simulink model "Scenario_13_CoDeSys"  (R2012b)
settings: Solver=ode3  StartTime=0.0  StopTime=inf  FixedStep=Sample_Time_Model  RelTol=1e-3
PreLoadFcn:
  | Variablen_Scenario13
InitFcn:
  | BT = randperm(9);
values from neighbouring files (symbols this model uses):
  Band_Geschwindigkeit = 1.47    [Variablen_Scenario13.m]
  Band_Sensor_Hell_2_Z = -6.5    [Variablen_Scenario13.m]
  Band_Sensor_Hell_3_Z = -10.36    [Variablen_Scenario13.m]
  Band_Sensor_Hell_4_Z = -14.64    [Variablen_Scenario13.m]
  Band_Sensor_Tolerance_Z = 0.2    [Variablen_Scenario13.m]
  Bauteil_Fallgeschwindigkeit = 0.4    [Variablen_Scenario13.m]
  Bauteil_Farbe_Metall = [0.8 0.8 0.8]    [Variablen_Scenario13.m]
  Bauteil_Farbe_Schwarz = [0.2 0.2 0.2]    [Variablen_Scenario13.m]
  Bauteil_Farbe_Weiss = [1 1 0.2]    [Variablen_Scenario13.m]
  Kran_Dauer_90_Grad = 5    [Variablen_Scenario13.m]
  Kran_Drehwinkel_90_Grad = 8050    [Variablen_Scenario13.m]
  Kran_Sensor_Position_Delta = 0.07    [Variablen_Scenario13.m]
  Sample_Time_Model = 0.05    [Variablen_Scenario13.m]
  Sample_Time_Simulation = 0.1    [Variablen_Scenario13.m]
  Sensor_Band_Metall_1 = -6.5    [Variablen_Scenario13.m]
  Sensor_Band_Metall_2 = -10.36    [Variablen_Scenario13.m]
libraries: simulink x557, vrlib x13, opclib x7, rtwinlib x1
(part 4 of 10)

== stateflow chart Scenario_13_CoDeSys/Signal Expander/Bauteil_4 ==
  state Stop1
  state Bauteil_Pos_2
  state Bauteil_Unten
  state Bauteil_Pos_4
    entry:
    BT_X_Achse = 5.75;
    BT_Y_Achse = 3.75;
    x =0;
  state Bauteil_Faellt_3
    during:
    BT_Y_Achse = Next_Pos_Minus_Min(BT_Y_Achse, Bauteil_Fallgeschwindigkeit, 0.7);
  state Drehen_Rechts_Runter [function]
    (default) -> (junction 322) : {BT_Y_Achse = Next_Pos_Minus_Min(BT_Y_Achse, Kran_Zyl_Schritt_Runter, 0.65);
        | x = x - Kran_Drehen_Schritt;
        | BT_Z_Achse = -3.5*sin(x);
        | BT_X_Achse = 3.5*cos(x);}
  state Drehen_Rechts_Hoch [function]
    (default) -> (junction 325) : {BT_Y_Achse = Next_Pos_Plus_Max(BT_Y_Achse, Kran_Zyl_Schritt_Hoch, 1.65);
        | x = x - Kran_Drehen_Schritt;
        | BT_Z_Achse = -3.5*sin(x);
        | BT_X_Achse = 3.5*cos(x);}
  state Bauteil_Lager_Vereinz_Ausfahren
    during:
    BT_X_Achse = BT_X_Achse - Lager_Vereinzler_Schritt_Aus;
  state Bauteil_Lager_Bereit
    entry: BT_Bereit = 1;
    BT_X_Achse = 3.5;
  state Drehen_Links_Runter [function]
    (default) -> (junction 319) : {BT_Y_Achse = Next_Pos_Minus_Min(BT_Y_Achse, Kran_Zyl_Schritt_Runter, 0.65);
        | x = x + Kran_Drehen_Schritt;
        | BT_Z_Achse = -3.5*sin(x);
        | BT_X_Achse = 3.5*cos(x);}
  state Drehen_Links_Hoch [function]
    (default) -> (junction 309) : {BT_Y_Achse = Next_Pos_Plus_Max(BT_Y_Achse, Kran_Zyl_Schritt_Hoch, 1.65);
        | x = x + Kran_Drehen_Schritt;
        | BT_Z_Achse = -3.5*sin(x);
        | BT_X_Achse = 3.5*cos(x);}
  state Ausgabe = Next_Pos_Plus_Max(Achse, Schrittgroesse, MaxWert) [function]
    (default) -> (junction 249) : {Naechste_Position = Achse + Schrittgroesse;}
    (junction 249) -> (junction 250) [order 1] : [Naechste_Position >= MaxWert]
    (junction 249) -> (junction 251) [order 2] : {Ausgabe = Naechste_Position;}
    (junction 250) -> (junction 252) : {Ausgabe = MaxWert;}
    (junction 252) -> (junction 251)
  state Bauteil_Pos_3
  state Bauteil_Kran_Hochheben_Bereit
    entry: BT_Bereit = 1;
    Kran_Sauger_BT = 1;
  state Bauteil_Faellt_2
    during:
    BT_Y_Achse = Next_Pos_Minus_Min(BT_Y_Achse, Bauteil_Fallgeschwindigkeit, 1.73);
  state Bauteil_Faellt
    during:
    BT_Y_Achse = Next_Pos_Minus_Min(BT_Y_Achse, Bauteil_Fallgeschwindigkeit, 2.75);
  state Ausgabe = Next_Pos_Minus_Min(Achse, Schrittgroesse, MinWert) [function]
    (default) -> (junction 268) : {Naechste_Position = Achse - Schrittgroesse;}
    (junction 268) -> (junction 269) [order 1] : [Naechste_Position <= MinWert]
    (junction 268) -> (junction 270) [order 2] : {Ausgabe = Naechste_Position;}
    (junction 269) -> (junction 271) : {Ausgabe = MinWert;}
    (junction 271) -> (junction 270)
  state Ausgabe = Lager_Y_Achse(Lager_Status, Pos_1, Pos_2, Pos_3) [function]
    (default) -> (junction 379)
    (junction 379) -> (junction 378) [order 3] : [Lager_Status == 2]
    (junction 379) -> (junction 380) [order 1] : [Lager_Status == 0]
    (junction 378) -> (junction 381) : {Ausgabe = Pos_3;}
    (junction 379) -> (junction 382) [order 2] : [Lager_Status == 1]
        | {Ausgabe = Pos_2;}
    (junction 380) -> (junction 383) : {Ausgabe = Pos_1;}
    (junction 381) -> (junction 382)
    (junction 383) -> (junction 382)
  state Bauteil_Stempel_Halterung_Einfahren
    during:
    BT_X_Achse = Next_Pos_Minus_Min(BT_X_Achse, Stempel_Halterung_Schritt_Ein, -4.6);
  state Bauteil_Kran_Runterlassen
    during:
    BT_Y_Achse = Next_Pos_Minus_Min(BT_Y_Achse, Kran_Zyl_Schritt_Runter, 0.65);
  state Bauteil_Kran_Hochheben
    during:
    BT_Y_Achse = Next_Pos_Plus_Max(BT_Y_Achse, Kran_Zyl_Schritt_Hoch, 1.65);
  state Bauteil_Faellt_Auf_Festen_Untergrund
  state Bauteil_Lost
  state Bauteil_Lager_1_Ende
    entry: BT_Y_Achse = Lager_Y_Achse(Lager_1_Status, -0.158, 0.037, 0.232);
    BT_Lager = 1;
  state Bauteil_Abgesetzt_Stempel
    entry: Kran_Sauger_BT = 0;
  state Bauteil_Kran_Zyl_Stop
  state Bauteil_Stempel_Halterung_Stop
  state Drop_Down
    entry: Kran_Sauger_BT = 0;
    during:
    BT_Y_Achse = BT_Y_Achse - 0.4;
  state Bauteil_Lager_1_Beginnt
    entry: BT_Rotation_1 = 0;
    BT_Rotation_2 = 0;
    BT_Rotation_3 = 1;
    BT_Rotation_4 = 0.2;
    during:
    BT_X_Achse = Next_Pos_Minus_Min(BT_X_Achse, Band_Zyl_1_Schritt, -6.5 + Lager_1_Status);
    BT_Y_Achse = BT_Y_Achse - (0.2 * Band_Zyl_1_Schritt);
  state Bauteil_Stempel_Halterung_Ausfahren
    during:
    BT_X_Achse = Next_Pos_Plus_Max(BT_X_Achse, Stempel_Halterung_Schritt_Aus, -3.4);
  note: Bei -2,8 beginnt in etwa die Schraege !!
  state Drehen_Links
    during:
    x = x + Kran_Drehen_Schritt;
    BT_Z_Achse = -3.5*sin(x);
    BT_X_Achse = 3.5*cos(x);
  state Bauteil_Band_Vor
    during:
    BT_Z_Achse = BT_Z_Achse - Band_Geschwindigkeit;
  state Bauteil_Lager_1_Schieben
    during:
    BT_X_Achse = Next_Pos_Minus_Min(BT_X_Achse, Band_Zyl_1_Schritt, -2.7);
  state Bauteil_Lager_2_Ende
    entry: BT_Y_Achse = Lager_Y_Achse(Lager_2_Status, -0.158, 0.037, 0.232);
    BT_Lager = 2;
  state Bauteil_Kran_Rot_Stop
  state Bauteil_Band_Stop
    entry: Kran_Sauger_BT = 0;
  state Drehen_Rechts
    during:
    x = x - Kran_Drehen_Schritt;
    BT_Z_Achse = -3.5*sin(x);
    BT_X_Achse = 3.5*cos(x);
  state Bauteil_Lager_2_Beginnt
    entry: BT_Rotation_1 = 0;
    BT_Rotation_2 = 0;
    BT_Rotation_3 = 1;
    BT_Rotation_4 = 0.2;
    during:
    BT_X_Achse = Next_Pos_Minus_Min(BT_X_Achse, Band_Zyl_2_Schritt, -6.5 + Lager_2_Status);
    BT_Y_Achse = BT_Y_Achse - (0.2 * Band_Zyl_2_Schritt);
  state Bauteil_Band_Zurueck
    during:
    BT_Z_Achse = BT_Z_Achse + Band_Geschwindigkeit;
  state Bauteil_Lager_2_Schieben
    during:
    BT_X_Achse = Next_Pos_Minus_Min(BT_X_Achse, Band_Zyl_2_Schritt, -2.7);
  state Bauteil_Kran_Runterlassen_Und_Drehen_Rechts
    entry:
    x = x - Kran_Drehen_Schritt;
    BT_Z_Achse = -3.5*sin(x);
    BT_X_Achse = 3.5*cos(x);
    during: Drehen_Rechts_Runter();
  state Bauteil_Lager_3_Beginnt
    entry: BT_Rotation_1 = -1;
    BT_Rotation_2 = 0;
    BT_Rotation_3 = 0;
    BT_Rotation_4 = 0.2;
    during:
    BT_Z_Achse = Next_Pos_Minus_Min(BT_Z_Achse, 1.5 * Band_Geschwindigkeit, -19.05 + Lager_3_Status);
    BT_Y_Achse = BT_Y_Achse - (1.5 * 0.2*Band_Geschwindigkeit);
  state Bauteil_Kran_Hochheben_Und_Drehen_Links
    entry:
    x = x + Kran_Drehen_Schritt;
    BT_Z_Achse = -3.5*sin(x);
    BT_X_Achse = 3.5*cos(x);
    during: Drehen_Links_Hoch();
  state Bauteil_Lager_3_Ende
    entry: BT_Y_Achse = Lager_Y_Achse(Lager_3_Status, -0.158, 0.037, 0.232);
    BT_Lager = 3;
  state Bauteil_Kran_Hochheben_Und_Drehen_Rechts
    entry:
    x = x - Kran_Drehen_Schritt;
    BT_Z_Achse = -3.5*sin(x);
    BT_X_Achse = 3.5*cos(x);
    during:Drehen_Rechts_Hoch();
  state Bauteil_Kran_Runterlassen_Und_Drehen_Links
    entry:
    x = x + Kran_Drehen_Schritt;
    BT_Z_Achse = -3.5*sin(x);
    BT_X_Achse = 3.5*cos(x);
    during: Drehen_Links_Runter();
  Bauteil_Faellt_Auf_Festen_Untergrund -> Bauteil_Abgesetzt_Stempel [order 2] : [Kran_Stellung_Stempel]
  (default) -> Bauteil_Pos_4
  Stop1 -> Bauteil_Lager_Vereinz_Ausfahren : [BT_X_Achse + Lager_X_Achse >= 5.1]
  Bauteil_Lager_Vereinz_Ausfahren -> Stop1 [order 2] : [BT_X_Achse + Lager_X_Achse < 5.1]
  Bauteil_Pos_2 -> Bauteil_Faellt_3 : [BT_3_Bereit && Lager_Ver_Eingefahren]
  Bauteil_Unten -> Bauteil_Lager_Vereinz_Ausfahren : [Lager_Ver_Ausfahren && (BT_X_Achse + Lager_X_Achse >= 5.1)]
  Bauteil_Faellt_2 -> Bauteil_Pos_2 : [BT_Y_Achse <= 1.73]
  Bauteil_Faellt_3 -> Bauteil_Unten : [BT_Y_Achse <= 0.7]
  Bauteil_Pos_4 -> Bauteil_Faellt : [BT_1_Bereit && Lager_Ver_Eingefahren]
  Bauteil_Lager_Vereinz_Ausfahren -> Bauteil_Lager_Bereit [order 1] : [Lager_Ver_Ausgefahren]
  Bauteil_Faellt_Auf_Festen_Untergrund -> Bauteil_Lager_Bereit [order 1] : [Kran_Stellung_Lager]
  Bauteil_Lager_Bereit -> Bauteil_Kran_Hochheben_Bereit : [Kran_Stellung_Lager && Kran_Sauger && Kran_Zyl_Unten]
  Bauteil_Stempel_Halterung_Stop -> Bauteil_Kran_Hochheben_Bereit [order 3] : [Kran_Stellung_Stempel && Kran_Sauger && Kran_Zyl_Unten]
  (junction 127) -> Bauteil_Kran_Hochheben_Bereit [order 2] : [Kran_Stellung_Lager && Kran_Sauger && Kran_Zyl_Unten]
  Bauteil_Faellt -> Bauteil_Pos_3 : [BT_Y_Achse <= 2.75]
  Bauteil_Kran_Hochheben_Bereit -> Bauteil_Kran_Hochheben : [Kran_Hochheben]
      | {BT_Bereit = 0;}
  Bauteil_Pos_3 -> Bauteil_Faellt_2 : [BT_2_Bereit && Lager_Ver_Eingefahren]
  Bauteil_Kran_Hochheben -> (junction 127) [order 3]
  Bauteil_Kran_Rot_Stop -> (junction 287) [order 4]
  (junction 287) -> Bauteil_Kran_Hochheben [order 2] : [Kran_Hochheben]
  (junction 287) -> Bauteil_Kran_Runterlassen [order 1] : [Kran_Runterlassen]
  Bauteil_Stempel_Halterung_Stop -> Bauteil_Stempel_Halterung_Einfahren [order 1] : [Stempel_Halterung_Einfahren]
  Bauteil_Stempel_Halterung_Einfahren -> Bauteil_Stempel_Halterung_Stop : [!Stempel_Halterung_Einfahren]
  Bauteil_Kran_Hochheben -> Bauteil_Kran_Runterlassen [order 1] : [Kran_Runterlassen]
  Bauteil_Kran_Runterlassen -> (junction 127) [order 2]
  Bauteil_Kran_Runterlassen -> (junction 162) [order 4]
  Bauteil_Kran_Zyl_Stop -> Bauteil_Kran_Runterlassen [order 3] : [Kran_Runterlassen]
  Bauteil_Kran_Runterlassen -> Bauteil_Kran_Zyl_Stop [order 3] : [Kran_Zyl_Unten]
  Bauteil_Kran_Runterlassen -> Bauteil_Kran_Hochheben [order 1] : [Kran_Hochheben]
  Drop_Down -> Bauteil_Faellt_Auf_Festen_Untergrund [order 2] : [(Kran_Stellung_Band || Kran_Stellung_Lager || Kran_Stellung_Stempel) && (BT_Y_Achse <= 0.65)]
  Drop_Down -> Bauteil_Lost [order 1] : [BT_Y_Achse <= -2]
  Bauteil_Kran_Hochheben -> (junction 162) [order 4]
  Bauteil_Kran_Hochheben -> Bauteil_Kran_Zyl_Stop [order 2] : [Kran_Zyl_Oben]
  Bauteil_Kran_Zyl_Stop -> Bauteil_Kran_Hochheben [order 2] : [Kran_Hochheben]
  Bauteil_Lager_1_Beginnt -> Bauteil_Lager_1_Ende : [BT_X_Achse <= (-6.5 + Lager_1_Status)]
  Bauteil_Abgesetzt_Stempel -> Bauteil_Stempel_Halterung_Stop
  Bauteil_Faellt_Auf_Festen_Untergrund -> Bauteil_Band_Stop [order 3] : [Kran_Stellung_Band]
  (junction 127) -> Drop_Down [order 1] : [!Kran_Sauger]
  Bauteil_Kran_Zyl_Stop -> (junction 127) [order 8]
  Bauteil_Kran_Zyl_Stop -> Bauteil_Abgesetzt_Stempel [order 6] : [Kran_Zyl_Unten && !Kran_Sauger && Kran_Stellung_Stempel]
  Drehen_Rechts -> Drop_Down [order 3] : [!Kran_Sauger]
  Bauteil_Stempel_Halterung_Ausfahren -> Bauteil_Stempel_Halterung_Stop : [!Stempel_Halterung_Ausfahren]
  Bauteil_Stempel_Halterung_Stop -> Bauteil_Stempel_Halterung_Ausfahren [order 2] : [Stempel_Halterung_Ausfahren]
  Bauteil_Kran_Rot_Stop -> Drop_Down [order 3] : [!Kran_Sauger]
  Drehen_Links -> Drop_Down [order 3] : [!Kran_Sauger]
  Bauteil_Kran_Zyl_Stop -> Drehen_Links [order 4] : [Kran_Drehen_Links]
  Bauteil_Kran_Zyl_Stop -> Drehen_Rechts [order 5] : [Kran_Drehen_Rechts]
  (junction 178) -> Bauteil_Kran_Zyl_Stop : [!Kran_Drehen_Rechts && !Kran_Drehen_Links]
  Bauteil_Kran_Zyl_Stop -> (junction 162) [order 1]
  Bauteil_Kran_Zyl_Stop -> Bauteil_Band_Stop [order 7] : [Kran_Zyl_Unten && !Kran_Sauger && Kran_Stellung_Band]
  Bauteil_Band_Stop -> Bauteil_Kran_Zyl_Stop [order 3] : [Kran_Zyl_Unten && Kran_Sauger && Kran_Stellung_Band && (-3.8 <= BT_Z_Achse) && (BT_Z_Achse <= -3.2) && (-0.3 <= BT_X_Achse) && (BT_X_Achse<= 0.3)]
  (junction 280) -> Drehen_Links [order 2] : [(Kran_Zyl_Unten || Kran_Zyl_Oben) && Kran_Drehen_Links]
      | {x = x + Kran_Drehen_Schritt;
      | BT_Z_Achse = -3.5*sin(x);
      | BT_X_Achse = 3.5*cos(x);}
  Drehen_Links -> Bauteil_Kran_Rot_Stop [order 2] : [!Kran_Drehen_Links]
  Bauteil_Lager_1_Schieben -> Bauteil_Lager_1_Beginnt : [BT_X_Achse <= -2.7]
  Bauteil_Kran_Rot_Stop -> Drehen_Links [order 1] : [Kran_Drehen_Links]
  Bauteil_Band_Vor -> (junction 135) [order 2]
  Drehen_Links -> (junction 162) [order 4]
  Drehen_Rechts -> Drehen_Links [order 1] : [Kran_Drehen_Links]
  Drehen_Links -> Drehen_Rechts [order 1] : [Kran_Drehen_Rechts]
  Bauteil_Band_Stop -> Bauteil_Band_Vor [order 1] : [Band_Vor]
  Bauteil_Band_Vor -> Bauteil_Band_Stop [order 1] : [!Band_Vor]
  (junction 135) -> Bauteil_Lager_1_Schieben [order 1] : [BT_Z_Achse <= -7.85 && BT_Z_Achse >= -8.65 && Band_Zyl_1_X_Achse >= -0.5]
  Bauteil_Lager_2_Beginnt -> Bauteil_Lager_2_Ende : [BT_X_Achse <= (-6.5 + Lager_2_Status)]
  (junction 280) -> Bauteil_Kran_Rot_Stop [order 3] : [Kran_Zyl_Unten || Kran_Zyl_Oben]
  Drehen_Rechts -> Bauteil_Kran_Rot_Stop [order 2] : [!Kran_Drehen_Rechts]
  Bauteil_Kran_Rot_Stop -> Drehen_Rechts [order 2] : [Kran_Drehen_Rechts]
  Bauteil_Band_Stop -> (junction 135) [order 4]
  (junction 135) -> Bauteil_Lager_2_Schieben [order 3] : [BT_Z_Achse <= -12.05 && BT_Z_Achse >= -12.85 && Band_Zyl_2_X_Achse >= -0.5]
  Bauteil_Band_Zurueck -> (junction 135) [order 2]
  (junction 135) -> Bauteil_Lager_3_Beginnt [order 2] : [BT_Z_Achse <= -14.6]
  Drehen_Rechts -> (junction 162) [order 4]
  Bauteil_Band_Zurueck -> Bauteil_Band_Stop [order 1] : [!Band_Zurueck]
  Bauteil_Band_Stop -> Bauteil_Band_Zurueck [order 2] : [Band_Zurueck]
  Bauteil_Kran_Runterlassen_Und_Drehen_Rechts -> (junction 178) [order 2]
  Bauteil_Kran_Hochheben_Und_Drehen_Links -> (junction 178) [order 2]
  Bauteil_Kran_Hochheben_Und_Drehen_Rechts -> (junction 178) [order 2]
  Bauteil_Kran_Runterlassen_Und_Drehen_Links -> (junction 178) [order 2]
  (junction 280) -> Drehen_Rechts [order 1] : [(Kran_Zyl_Unten || Kran_Zyl_Oben) && Kran_Drehen_Rechts]
      | {x = x - Kran_Drehen_Schritt;
      | BT_Z_Achse = -3.5*sin(x);
      | BT_X_Achse = 3.5*cos(x);}
  (junction 172) -> (junction 280)
  (junction 162) -> Bauteil_Kran_Runterlassen_Und_Drehen_Rechts [order 4] : [Kran_Drehen_Rechts && Kran_Runterlassen]
  (junction 162) -> Bauteil_Kran_Hochheben_Und_Drehen_Rechts [order 2] : [Kran_Drehen_Rechts && Kran_Hochheben]
  (junction 162) -> Bauteil_Kran_Hochheben_Und_Drehen_Links [order 1] : [Kran_Drehen_Links  && Kran_Hochheben]
  (junction 162) -> Bauteil_Kran_Runterlassen_Und_Drehen_Links [order 3] : [Kran_Drehen_Links  && Kran_Runterlassen]
  Bauteil_Lager_2_Schieben -> Bauteil_Lager_2_Beginnt : [BT_X_Achse <= -2.7]
  Bauteil_Kran_Runterlassen_Und_Drehen_Rechts -> (junction 172) [order 1]
  Bauteil_Lager_3_Beginnt -> Bauteil_Lager_3_Ende : [BT_Z_Achse <= (-19.05 + Lager_3_Status)]
  Bauteil_Kran_Hochheben_Und_Drehen_Rechts -> Bauteil_Kran_Runterlassen_Und_Drehen_Rechts [order 3] : [Kran_Drehen_Rechts  && Kran_Runterlassen]
  Bauteil_Kran_Runterlassen_Und_Drehen_Rechts -> Bauteil_Kran_Hochheben_Und_Drehen_Rechts [order 3] : [Kran_Drehen_Rechts  && Kran_Hochheben]
  Bauteil_Kran_Hochheben_Und_Drehen_Rechts -> (junction 172) [order 1]
  Bauteil_Kran_Hochheben_Und_Drehen_Links -> (junction 172) [order 1]
  Bauteil_Kran_Hochheben_Und_Drehen_Links -> Bauteil_Kran_Runterlassen_Und_Drehen_Links [order 3] : [Kran_Drehen_Links  && Kran_Runterlassen]
  Bauteil_Kran_Runterlassen_Und_Drehen_Links -> Bauteil_Kran_Hochheben_Und_Drehen_Links [order 3] : [Kran_Drehen_Links  && Kran_Hochheben]
  Bauteil_Kran_Runterlassen_Und_Drehen_Links -> (junction 172) [order 1]
  data: Achse function_input double; Schrittgroesse function_input double; MaxWert function_input double; Ausgabe function_output double; Achse function_input double; Schrittgroesse function_input double; MinWert function_input double; Ausgabe function_output double; Lager_Status function_input double; Pos_1 function_input double; Pos_2 function_input double; Ausgabe function_output double; Pos_3 function_input double; BT_Y_Achse output double; BT_Lager output double; Kran_Sauger_BT output double; BT_Bereit output double; BT_X_Achse output double; BT_Z_Achse output double; x local double; Lager_X_Achse input; Lager_Ver_Eingefahren input; Lager_Ver_Ausgefahren input; Kran_Stellung_Lager input; Kran_Stellung_Band input; Kran_Stellung_Stempel input; Kran_Zyl_Oben input; Kran_Zyl_Unten input; Kran_Sauger input; Kran_Hochheben input; Kran_Runterlassen input; Kran_Drehen_Links input; Kran_Drehen_Rechts input; Stempel_Halterung_Ausfahren input; Stempel_Halterung_Einfahren input; Band_Vor input; Band_Zurueck input; Band_Zyl_1_X_Achse input; Band_Zyl_2_X_Achse input; BT_Rotation_1 output double; BT_Rotation_2 output double; BT_Rotation_3 output double; BT_Rotation_4 output double; Lager_Ver_Ausfahren input; Lager_Vereinzler_Schritt_Aus input; Kran_Zyl_Schritt_Hoch input; Kran_Zyl_Schritt_Runter input; Kran_Drehen_Schritt input; Stempel_Halterung_Schritt_Aus input; Stempel_Halterung_Schritt_Ein input; Band_Zyl_1_Schritt input; Band_Zyl_2_Schritt input double; Band_Geschwindigkeit input; Bauteil_Fallgeschwindigkeit input double; Lager_1_Status input; Lager_2_Status input; Lager_3_Status input; Naechste_Position local double; BT_1_Bereit input; BT_2_Bereit input; BT_3_Bereit input

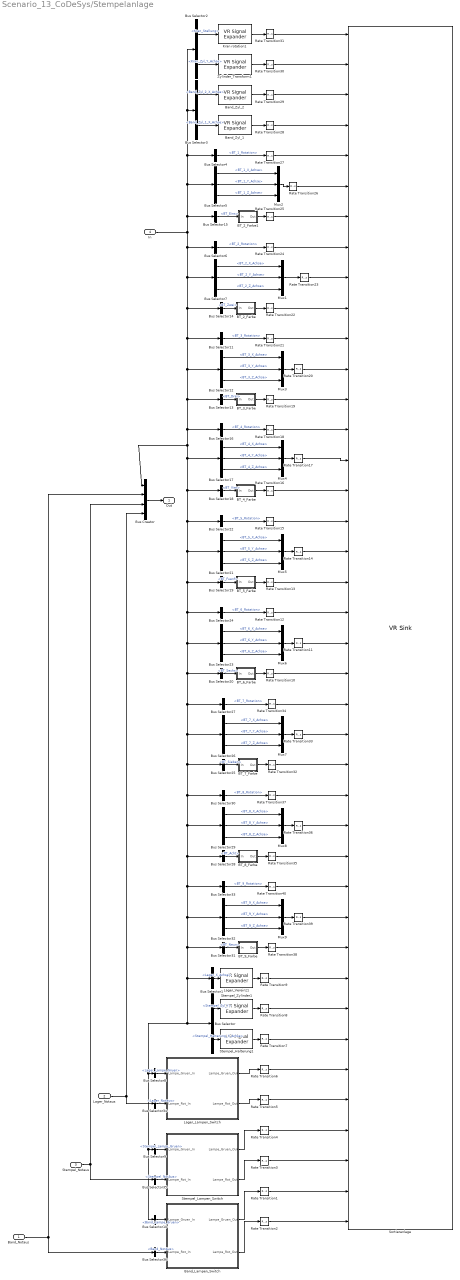
== system Scenario_13_CoDeSys/Stempelanlage ==
  Band_Notaus : Inport
  Lager_Notaus : Inport  Port=2
  Stempel_Notaus : Inport  Port=3
  In : Inport  Port=4
  BT_2_Farbe : Subsystem
  BT_2_Farbe1 : Subsystem
  BT_3_Farbe : Subsystem
  BT_4_Farbe : Subsystem
  BT_5_Farbe : Subsystem
  BT_6_Farbe : Subsystem
  BT_7_Farbe : Subsystem
  BT_8_Farbe : Subsystem
  BT_9_Farbe : Subsystem
  Band_Lampen_Switch : Subsystem
  Band_Zyl_1 : vrlib/VR Signal Expander  outwidth=3  outidx=2
  Band_Zyl_2 : vrlib/VR Signal Expander  outwidth=3  outidx=2
  Bus Creator : BusCreator
  Bus Selector : BusSelector  OutputSignals=Bauteil.Stempelanlage_BT.Stempelanlage.Stempel.Stempel_Zyl.Stempel_Zyl_Y,Bauteil.Stempelanlage_BT.Stempelanlage.Stempel.Stempel_Halterung_X_Achse
  Bus Selector1 : BusSelector  OutputSignals=Bauteil.Stempelanlage_BT.Stempelanlage.Lager.Lager_X_Achse
  Bus Selector10 : BusSelector  OutputSignals=Eingaenge.Band.Band_Lampe_Gruen
  Bus Selector11 : BusSelector  OutputSignals=Bauteil.Stempelanlage_BT.Bauteil_3.BT_3_Rotation
  Bus Selector12 : BusSelector  OutputSignals=Bauteil.Stempelanlage_BT.Bauteil_3.BT_3_X_Achse,Bauteil.Stempelanlage_BT.Bauteil_3.BT_3_Y_Achse,Bauteil.Stempelanlage_BT.Bauteil_3.BT_3_Z_Achse
  Bus Selector13 : BusSelector  OutputSignals=Eingaenge.Bauteile.BT_Drei
  Bus Selector14 : BusSelector  OutputSignals=Eingaenge.Bauteile.BT_Zwei
  Bus Selector15 : BusSelector  OutputSignals=Eingaenge.Bauteile.BT_Eins
  Bus Selector16 : BusSelector  OutputSignals=Bauteil.Stempelanlage_BT.Bauteil_4.BT_4_Rotation
  Bus Selector17 : BusSelector  OutputSignals=Bauteil.Stempelanlage_BT.Bauteil_4.BT_4_X_Achse,Bauteil.Stempelanlage_BT.Bauteil_4.BT_4_Y_Achse,Bauteil.Stempelanlage_BT.Bauteil_4.BT_4_Z_Achse
  Bus Selector18 : BusSelector  OutputSignals=Eingaenge.Bauteile.BT_Vier
  Bus Selector19 : BusSelector  OutputSignals=Eingaenge.Bauteile.BT_Fuenf
  Bus Selector2 : BusSelector  OutputSignals=Bauteil.Stempelanlage_BT.Stempelanlage.Kran.Kran_Stellung,Bauteil.Stempelanlage_BT.Stempelanlage.Kran.Kran_Zyl.Kran_Zyl_Y_Achse
  Bus Selector20 : BusSelector  OutputSignals=Eingaenge.Bauteile.BT_Sechs
  Bus Selector21 : BusSelector  OutputSignals=Bauteil.Stempelanlage_BT.Bauteil_5.BT_5_X_Achse,Bauteil.Stempelanlage_BT.Bauteil_5.BT_5_Y_Achse,Bauteil.Stempelanlage_BT.Bauteil_5.BT_5_Z_Achse
  Bus Selector22 : BusSelector  OutputSignals=Bauteil.Stempelanlage_BT.Bauteil_5.BT_5_Rotation
  Bus Selector23 : BusSelector  OutputSignals=Bauteil.Stempelanlage_BT.Bauteil_6.BT_6_X_Achse,Bauteil.Stempelanlage_BT.Bauteil_6.BT_6_Y_Achse,Bauteil.Stempelanlage_BT.Bauteil_6.BT_6_Z_Achse
  Bus Selector24 : BusSelector  OutputSignals=Bauteil.Stempelanlage_BT.Bauteil_6.BT_6_Rotation
  Bus Selector25 : BusSelector  OutputSignals=Eingaenge.Bauteile.BT_Sieben
  Bus Selector26 : BusSelector  OutputSignals=Bauteil.Stempelanlage_BT.Bauteil_7.BT_7_X_Achse,Bauteil.Stempelanlage_BT.Bauteil_7.BT_7_Y_Achse,Bauteil.Stempelanlage_BT.Bauteil_7.BT_7_Z_Achse
  Bus Selector27 : BusSelector  OutputSignals=Bauteil.Stempelanlage_BT.Bauteil_7.BT_7_Rotation
  Bus Selector28 : BusSelector  OutputSignals=Eingaenge.Bauteile.BT_Acht
  Bus Selector29 : BusSelector  OutputSignals=Bauteil.Stempelanlage_BT.Bauteil_8.BT_8_X_Achse,Bauteil.Stempelanlage_BT.Bauteil_8.BT_8_Y_Achse,Bauteil.Stempelanlage_BT.Bauteil_8.BT_8_Z_Achse
  Bus Selector3 : BusSelector  OutputSignals=Bauteil.Stempelanlage_BT.Stempelanlage.Band.Band_Zyl_2_X_Achse,Bauteil.Stempelanlage_BT.Stempelanlage.Band.Band_Zyl_1_X_Achse
  Bus Selector30 : BusSelector  OutputSignals=Bauteil.Stempelanlage_BT.Bauteil_8.BT_8_Rotation
  Bus Selector31 : BusSelector  OutputSignals=Eingaenge.Bauteile.BT_Neun
  Bus Selector32 : BusSelector  OutputSignals=Bauteil.Stempelanlage_BT.Bauteil_9.BT_9_X_Achse,Bauteil.Stempelanlage_BT.Bauteil_9.BT_9_Y_Achse,Bauteil.Stempelanlage_BT.Bauteil_9.BT_9_Z_Achse
  Bus Selector33 : BusSelector  OutputSignals=Bauteil.Stempelanlage_BT.Bauteil_9.BT_9_Rotation
  Bus Selector34 : BusSelector  OutputSignals=Lager_Notaus
  Bus Selector35 : BusSelector  OutputSignals=Stempel_NotAus
  Bus Selector36 : BusSelector  OutputSignals=Band_NotAus
  Bus Selector4 : BusSelector  OutputSignals=Bauteil.Stempelanlage_BT.Bauteil_1.BT_1_Rotation
  Bus Selector5 : BusSelector  OutputSignals=Bauteil.Stempelanlage_BT.Bauteil_1.BT_1_X_Achse,Bauteil.Stempelanlage_BT.Bauteil_1.BT_1_Y_Achse,Bauteil.Stempelanlage_BT.Bauteil_1.BT_1_Z_Achse
  Bus Selector6 : BusSelector  OutputSignals=Bauteil.Stempelanlage_BT.Bauteil_2.BT_2_Rotation
  Bus Selector7 : BusSelector  OutputSignals=Bauteil.Stempelanlage_BT.Bauteil_2.BT_2_X_Achse,Bauteil.Stempelanlage_BT.Bauteil_2.BT_2_Y_Achse,Bauteil.Stempelanlage_BT.Bauteil_2.BT_2_Z_Achse
  Bus Selector8 : BusSelector  OutputSignals=Eingaenge.Lager.Lager_Lampe_Gruen
  Bus Selector9 : BusSelector  OutputSignals=Eingaenge.Stempel.Stempel_Lampe_Gruen
  Kran rotation1 : vrlib/VR Signal Expander  outwidth=4  outidx=4
  Lager_Lampen_Switch : Subsystem
  Lager_Vereinz1 : vrlib/VR Signal Expander  outwidth=3  outidx=2
  Mux{1..9} (9 alike) : Mux  Inputs=3
  Rate Transition{1..40} (40 alike) : RateTransition
  Sortieranlage : vrlib/VR Sink  InstantiateOnLoad=on  SampleTime=Sample_Time_Simulation  ViewEnable=on  RemoteChange=off  RemoteView=off  FieldsWritten=Kran.rotation.4.1.1.double#Kran_Zyl.translation.3.1.1.double#Foerd_Vereinz_2.translation.3.1.1.double#Foerd_Vereinz_1.translation.3.1.1.double#Bauteil_1.rotation.4.1.1.double#Bauteil_1.translation.3.1.1.double#B1_Material.diffuseColor.3.1.1.double#Bauteil_2.rotation.4.1.1.double#Bauteil_2.translation.3.1.1.double#B2_Material.diffuseColor.3.1.1.double#Bauteil_3.rotation.4.1.1.double#Bauteil_3.translation.3.1.1.double#B3_Material.diffuseColor.3.1.1.double#Bauteil_4.rotation.4.1.1.double#Bauteil_4.translation.3.1.1.double#B4_Material.diffuseColor.3.1.1.double#Bauteil_5.rotation.4.1.1.double#Bauteil_5.translation.3.1.1.double#B5_Material.diffuseColor.3.1.1.double#Bauteil_6.rotation.4.1.1.double#Bauteil_6.translation.3.1.1.double#B6_Material.diffuseColor.3.1.1.double#Bauteil_7.rotation.4.1.1.double#Bauteil_7.translation.3.1.1.double#B7_Material.diffuseColor.3.1.1.double#Bauteil_8.rotation.4.1.1.double#Bauteil_8.translation.3.1.1.double#B8_Material.diffuseColor.3.1.1.double#Bauteil_9.rotation.4.1.1.double#Bauteil_9.translation.3.1.1.double#B9_Material.diffuseColor.3.1.1.double#Lager_Vereinz_Translation.translation.3.1.1.double#Stempel_Zylinder.translation.3.1.1.double#Stempel_Halterung.translation.3.1.1.double#Lampe_1.diffuseColor.3.1.1.double#Lampe_2.diffuseColor.3.1.1.double#Lampe_3.diffuseColor.3.1.1.double#Lampe_4.diffuseColor.3.1.1.double#Lampe_5.diffuseColor.3.1.1.double#Lampe_6.diffuseColor.3.1.1.double  WorldFileName=Visu_Sz_13.wrl  AutoView=on  VideoDimensions=[]  AllowVariableSize=off  FigureProperties="{'Position', 'Name', 'Viewpoint', 'CameraBound', 'CameraDirection', 'CameraPosition', 'CameraUpVector', 'ZoomFactor', 'Antialiasing', 'Headlight', 'Lighting', 'NavPanel', 'StatusBar', 'ToolBar', 'Textures', 'Transparency', 'Triad', 'Wireframe', 'NavZones', 'NavMode', 'NavSpeed', 'CaptureFileFormat', 'CaptureFileName', 'Record2DCompressMethod', 'Record2DCompressQuality', 'Record2D', 'Record2DFileName', 'Record2DFPS'; [5.0000000000000000e+00   9.2000000000000000e+01   5.7600000000000000e+02   3.8000000000000000e+02], '', '', 'on', [0.0000000000000000e+00   0.0000000000000000e+00  -1.0000000000000000e+00], [0.0000000000000000e+00   0.0000000000000000e+00   1.0000000000000000e+01], [0.0000000000000000e+00   1.0000000000000000e+00   0.0000000000000000e+00], [1.0000000000000000e+00], 'on', 'off', 'on', 'halfbar', 'on', 'on', 'on', 'on', 'none', 'off', 'off', 'examine', 'normal', 'tif', '%f_anim_%n.tif', 'auto', [7.5000000000000000e+01], 'off', '%f_anim_%n.avi', [1.5000000000000000e+01]}"
  Stempel_Halterung1 : vrlib/VR Signal Expander  outwidth=3  outidx=2
  Stempel_Lampen_Switch : Subsystem
  Stempel_Zylinder1 : vrlib/VR Signal Expander  outwidth=3  outidx=2
  Zylinder_Transform1 : vrlib/VR Signal Expander  outwidth=3  outidx=2
  Out : Outport
  wires:
  Bus Selector/1 -> Stempel_Zylinder1/1  "<Stempel_Zyl_Y>"
  Bus Selector/2 -> Stempel_Halterung1/1  "<Stempel_Halterung_X_Achse>"
  Bus Selector1/1 -> Lager_Vereinz1/1  "<Lager_X_Achse>"
  Bus Selector2/1 -> Kran rotation1/1  "<Kran_Stellung>"
  Bus Selector3/2 -> Band_Zyl_1/1  "<Band_Zyl_1_X_Achse>"
  Bus Selector3/1 -> Band_Zyl_2/1  "<Band_Zyl_2_X_Achse>"
  Bus Selector2/2 -> Zylinder_Transform1/1  "<Kran_Zyl_Y_Achse>"
  Bus Selector5/1 -> Mux2/1  "<BT_1_X_Achse>"
  Bus Selector5/2 -> Mux2/2  "<BT_1_Y_Achse>"
  Bus Selector7/1 -> Mux1/1  "<BT_2_X_Achse>"
  Bus Selector7/2 -> Mux1/2  "<BT_2_Y_Achse>"
  Lager_Notaus/1 -> Bus Selector34/1, Bus Creator/4
  Bus Creator/1 -> Out/1
  Bus Selector12/1 -> Mux3/1  "<BT_3_X_Achse>"
  Bus Selector12/2 -> Mux3/2  "<BT_3_Y_Achse>"
  Bus Selector13/1 -> BT_3_Farbe/1(In)  "<BT_Drei>"
  Bus Selector14/1 -> BT_2_Farbe/1(In)  "<BT_Zwei>"
  Bus Selector15/1 -> BT_2_Farbe1/1(In)  "<BT_Eins>"
  Kran rotation1/1 -> Rate Transition31/1
  Zylinder_Transform1/1 -> Rate Transition30/1
  Band_Zyl_2/1 -> Rate Transition29/1
  Band_Zyl_1/1 -> Rate Transition28/1
  Bus Selector4/1 -> Rate Transition27/1  "<BT_1_Rotation>"
  Mux2/1 -> Rate Transition26/1
  BT_2_Farbe1/1(Out) -> Rate Transition25/1
  Bus Selector6/1 -> Rate Transition24/1  "<BT_2_Rotation>"
  Mux1/1 -> Rate Transition23/1
  BT_2_Farbe/1(Out) -> Rate Transition22/1
  Bus Selector11/1 -> Rate Transition21/1  "<BT_3_Rotation>"
  Mux3/1 -> Rate Transition20/1
  BT_3_Farbe/1(Out) -> Rate Transition19/1
  Lager_Vereinz1/1 -> Rate Transition9/1
  Stempel_Zylinder1/1 -> Rate Transition8/1
  Stempel_Halterung1/1 -> Rate Transition7/1
  Lager_Lampen_Switch/1(Lampe_Gruen_Out) -> Rate Transition6/1
  Lager_Lampen_Switch/2(Lampe_Rot_Out) -> Rate Transition5/1
  Bus Selector16/1 -> Rate Transition18/1  "<BT_4_Rotation>"
  Bus Selector17/1 -> Mux4/1  "<BT_4_X_Achse>"
  Bus Selector17/2 -> Mux4/2  "<BT_4_Y_Achse>"
  Mux4/1 -> Rate Transition17/1
  BT_4_Farbe/1(Out) -> Rate Transition16/1
  BT_5_Farbe/1(Out) -> Rate Transition13/1
  BT_6_Farbe/1(Out) -> Rate Transition10/1
  Bus Selector18/1 -> BT_4_Farbe/1(In)  "<BT_Vier>"
  Bus Selector19/1 -> BT_5_Farbe/1(In)  "<BT_Fuenf>"
  Bus Selector20/1 -> BT_6_Farbe/1(In)  "<BT_Sechs>"
  Bus Selector21/1 -> Mux5/1  "<BT_5_X_Achse>"
  Bus Selector21/2 -> Mux5/2  "<BT_5_Y_Achse>"
  Mux5/1 -> Rate Transition14/1
  Bus Selector22/1 -> Rate Transition15/1  "<BT_5_Rotation>"
  Bus Selector23/1 -> Mux6/1  "<BT_6_X_Achse>"
  Bus Selector23/2 -> Mux6/2  "<BT_6_Y_Achse>"
  Mux6/1 -> Rate Transition11/1
  Bus Selector24/1 -> Rate Transition12/1  "<BT_6_Rotation>"
  Band_Notaus/1 -> Bus Creator/2, Bus Selector36/1
  Band_Lampen_Switch/1(Lampe_Gruen_Out) -> Rate Transition1/1
  Band_Lampen_Switch/2(Lampe_Rot_Out) -> Rate Transition2/1
  Stempel_Notaus/1 -> Bus Selector35/1, Bus Creator/3
  Stempel_Lampen_Switch/1(Lampe_Gruen_Out) -> Rate Transition4/1
  Stempel_Lampen_Switch/2(Lampe_Rot_Out) -> Rate Transition3/1
  BT_7_Farbe/1(Out) -> Rate Transition32/1
  Bus Selector25/1 -> BT_7_Farbe/1(In)  "<BT_Sieben>"
  Bus Selector26/1 -> Mux7/1  "<BT_7_X_Achse>"
  Bus Selector26/2 -> Mux7/2  "<BT_7_Y_Achse>"
  Mux7/1 -> Rate Transition33/1
  Bus Selector27/1 -> Rate Transition34/1  "<BT_7_Rotation>"
  BT_8_Farbe/1(Out) -> Rate Transition35/1
  Bus Selector28/1 -> BT_8_Farbe/1(In)  "<BT_Acht>"
  Bus Selector29/1 -> Mux8/1  "<BT_8_X_Achse>"
  Bus Selector29/2 -> Mux8/2  "<BT_8_Y_Achse>"
  Mux8/1 -> Rate Transition36/1
  Bus Selector30/1 -> Rate Transition37/1  "<BT_8_Rotation>"
  BT_9_Farbe/1(Out) -> Rate Transition38/1
  Bus Selector31/1 -> BT_9_Farbe/1(In)  "<BT_Neun>"
  Bus Selector32/1 -> Mux9/1  "<BT_9_X_Achse>"
  Bus Selector32/2 -> Mux9/2  "<BT_9_Y_Achse>"
  In/1 -> Bus Selector15/1, Bus Selector2/1, Bus Selector3/1, Bus Selector4/1, Bus Selector5/1, Bus Selector27/1, Bus Selector26/1, Bus Selector25/1, Bus Selector30/1, Bus Selector29/1, Bus Selector28/1, Bus Selector33/1, Bus Selector32/1, Bus Selector31/1, Bus Selector9/1, Bus Selector10/1, Bus Selector8/1, Bus Selector/1, Bus Selector1/1, Bus Selector20/1, Bus Selector23/1, Bus Selector24/1, Bus Selector19/1, Bus Selector21/1, Bus Selector22/1, Bus Selector18/1, Bus Selector17/1, Bus Creator/1, Bus Selector16/1, Bus Selector13/1, Bus Selector12/1, Bus Selector11/1, Bus Selector14/1, Bus Selector7/1, Bus Selector6/1
  Mux9/1 -> Rate Transition39/1
  Bus Selector33/1 -> Rate Transition40/1  "<BT_9_Rotation>"
  Bus Selector8/1 -> Lager_Lampen_Switch/1(Lampe_Gruen_In)  "<Lager_Lampe_Gruen>"
  Bus Selector9/1 -> Stempel_Lampen_Switch/1(Lampe_Gruen_In)  "<Stempel_Lampe_Gruen>"
  Bus Selector10/1 -> Band_Lampen_Switch/1(Lampe_Gruen_In)  "<Band_Lampe_Gruen>"
  Bus Selector34/1 -> Lager_Lampen_Switch/2(Lampe_Rot_In)  "<Lager_Notaus>"
  Bus Selector35/1 -> Stempel_Lampen_Switch/2(Lampe_Rot_In)  "<Stempel_NotAus>"
  Bus Selector36/1 -> Band_Lampen_Switch/2(Lampe_Rot_In)  "<Band_NotAus>"
  Bus Selector7/3 -> Mux1/3  "<BT_2_Z_Achse>"
  Bus Selector12/3 -> Mux3/3  "<BT_3_Z_Achse>"
  Bus Selector17/3 -> Mux4/3  "<BT_4_Z_Achse>"
  Bus Selector21/3 -> Mux5/3  "<BT_5_Z_Achse>"
  Bus Selector23/3 -> Mux6/3  "<BT_6_Z_Achse>"
  Bus Selector26/3 -> Mux7/3  "<BT_7_Z_Achse>"
  Bus Selector29/3 -> Mux8/3  "<BT_8_Z_Achse>"
  Bus Selector32/3 -> Mux9/3  "<BT_9_Z_Achse>"
  Bus Selector5/3 -> Mux2/3  "<BT_1_Z_Achse>"
  Rate Transition31/1 -> Sortieranlage/1
  Rate Transition30/1 -> Sortieranlage/2
  Rate Transition29/1 -> Sortieranlage/3
  Rate Transition28/1 -> Sortieranlage/4
  Rate Transition27/1 -> Sortieranlage/5
  Rate Transition26/1 -> Sortieranlage/6
  Rate Transition25/1 -> Sortieranlage/7
  Rate Transition24/1 -> Sortieranlage/8
  Rate Transition23/1 -> Sortieranlage/9
  Rate Transition22/1 -> Sortieranlage/10
  Rate Transition21/1 -> Sortieranlage/11
  Rate Transition20/1 -> Sortieranlage/12
  Rate Transition19/1 -> Sortieranlage/13
  Rate Transition18/1 -> Sortieranlage/14
  Rate Transition17/1 -> Sortieranlage/15
  Rate Transition16/1 -> Sortieranlage/16
  Rate Transition15/1 -> Sortieranlage/17
  Rate Transition14/1 -> Sortieranlage/18
  Rate Transition13/1 -> Sortieranlage/19
  Rate Transition12/1 -> Sortieranlage/20
  Rate Transition11/1 -> Sortieranlage/21
  Rate Transition10/1 -> Sortieranlage/22
  Rate Transition34/1 -> Sortieranlage/23
  Rate Transition33/1 -> Sortieranlage/24
  Rate Transition32/1 -> Sortieranlage/25
  Rate Transition37/1 -> Sortieranlage/26
  Rate Transition36/1 -> Sortieranlage/27
  Rate Transition35/1 -> Sortieranlage/28
  Rate Transition40/1 -> Sortieranlage/29
  Rate Transition39/1 -> Sortieranlage/30
  Rate Transition38/1 -> Sortieranlage/31
  Rate Transition9/1 -> Sortieranlage/32
  Rate Transition8/1 -> Sortieranlage/33
  Rate Transition7/1 -> Sortieranlage/34
  Rate Transition6/1 -> Sortieranlage/35
  Rate Transition5/1 -> Sortieranlage/36
  Rate Transition4/1 -> Sortieranlage/37
  Rate Transition3/1 -> Sortieranlage/38
  Rate Transition1/1 -> Sortieranlage/39
  Rate Transition2/1 -> Sortieranlage/40

== system Scenario_13_CoDeSys/Inputs/Subsystem1 ==
  BT_Input_and_Shuffle_Button : Subsystem
  Demux : Demux  Outputs=9
  Subsystem : Subsystem
  Subsystem1 : Subsystem
  Subsystem2 : Subsystem
  Subsystem3 : Subsystem
  Subsystem4 : Subsystem
  Subsystem5 : Subsystem
  Subsystem6 : Subsystem
  Subsystem7 : Subsystem
  Subsystem8 : Subsystem
  BT1 : Outport
  BT2 : Outport  Port=2
  BT3 : Outport  Port=3
  BT4 : Outport  Port=4
  BT5 : Outport  Port=5
  BT6 : Outport  Port=6
  BT7 : Outport  Port=7
  BT8 : Outport  Port=8
  BT9 : Outport  Port=9
  wires:
  BT_Input_and_Shuffle_Button/1(Out) -> Demux/1
  Demux/1 -> Subsystem/1(BT_In)
  Demux/3 -> Subsystem2/1(BT_In)
  Demux/4 -> Subsystem3/1(BT_In)
  Demux/5 -> Subsystem4/1(BT_In)
  Demux/6 -> Subsystem5/1(BT_In)
  Demux/7 -> Subsystem6/1(BT_In)
  Demux/8 -> Subsystem7/1(BT_In)
  Demux/9 -> Subsystem8/1(BT_In)
  Subsystem/1(BT_Out) -> BT1/1
  Subsystem1/1(BT_Out) -> BT2/1
  Demux/2 -> Subsystem1/1(BT_In)
  Subsystem2/1(BT_Out) -> BT3/1
  Subsystem3/1(BT_Out) -> BT4/1
  Subsystem4/1(BT_Out) -> BT5/1
  Subsystem5/1(BT_Out) -> BT6/1
  Subsystem6/1(BT_Out) -> BT7/1
  Subsystem7/1(BT_Out) -> BT8/1
  Subsystem8/1(BT_Out) -> BT9/1

== system Scenario_13_CoDeSys/Sensoren/Kran_Sauger_BT ==
  BT_1 : Inport
  BT_2 : Inport  Port=2
  BT_3 : Inport  Port=3
  BT_4 : Inport  Port=4
  BT_5 : Inport  Port=5
  BT_6 : Inport  Port=6
  BT_7 : Inport  Port=7
  BT_8 : Inport  Port=8
  BT_9 : Inport  Port=9
  Display{,1..9} (10 alike) : Display
  Logical Operator1 : Logic  Operator=OR  Inputs=9  AllPortsSameDT=off  OutDataTypeStr=boolean
  Kran_Sauger_BT : Outport
  wires:
  Logical Operator1/1 -> Display9/1, Kran_Sauger_BT/1
  BT_1/1 -> Display/1, Logical Operator1/1
  BT_2/1 -> Display1/1, Logical Operator1/2
  BT_3/1 -> Display2/1, Logical Operator1/3
  BT_4/1 -> Display3/1, Logical Operator1/4
  BT_5/1 -> Display4/1, Logical Operator1/5
  BT_7/1 -> Display6/1, Logical Operator1/7
  BT_8/1 -> Display7/1, Logical Operator1/8
  BT_9/1 -> Display8/1, Logical Operator1/9
  BT_6/1 -> Display5/1, Logical Operator1/6

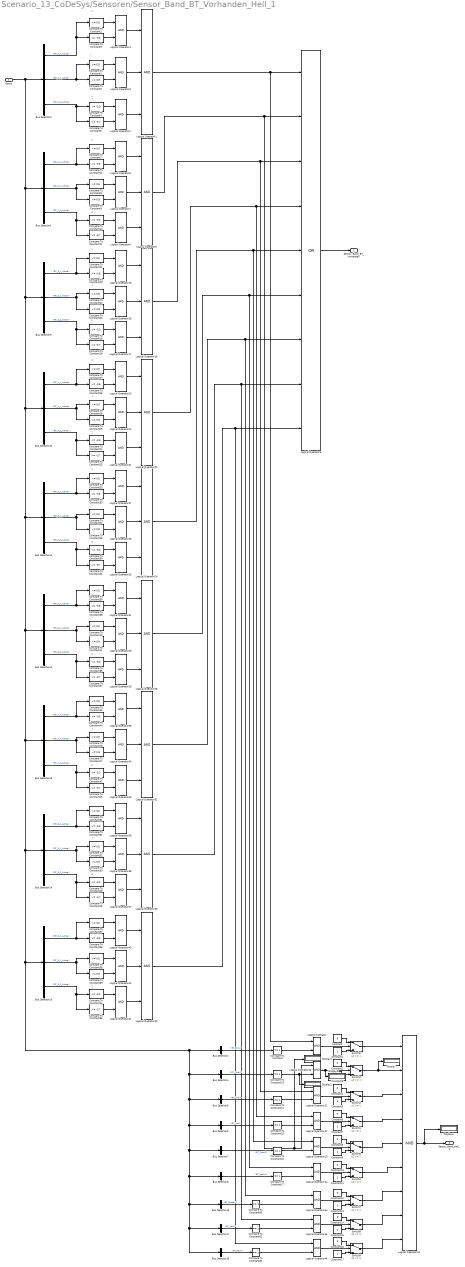
== system Scenario_13_CoDeSys/Sensoren/Sensor_Band_BT_Vorhanden_Hell_1 ==
  note: Z
  note: Y
  note: X
  note: Z
  note: Y
  note: X
  note: Z
  note: Y
  note: X
  note: Z
  note: Y
  note: X
  note: Z
  note: Y
  note: X
  note: Z
  note: Y
  note: Z
  note: Y
  note: Z
  note: Y
  note: Z
  note: Y
  Inputs : Inport
  Bus Selector1 : BusSelector  OutputSignals=Bauteil.Stempelanlage_BT.Bauteil_2.BT_2_X_Achse,Bauteil.Stempelanlage_BT.Bauteil_2.BT_2_Y_Achse,Bauteil.Stempelanlage_BT.Bauteil_2.BT_2_Z_Achse
  Bus Selector10 : BusSelector  OutputSignals=Bauteil.Stempelanlage_BT.Bauteil_4.BT_4_X_Achse,Bauteil.Stempelanlage_BT.Bauteil_4.BT_4_Y_Achse,Bauteil.Stempelanlage_BT.Bauteil_4.BT_4_Z_Achse
  Bus Selector11 : BusSelector  OutputSignals=Bauteil.Stempelanlage_BT.Bauteil_5.BT_5_X_Achse,Bauteil.Stempelanlage_BT.Bauteil_5.BT_5_Y_Achse,Bauteil.Stempelanlage_BT.Bauteil_5.BT_5_Z_Achse
  Bus Selector12 : BusSelector  OutputSignals=Bauteil.Stempelanlage_BT.Bauteil_6.BT_6_X_Achse,Bauteil.Stempelanlage_BT.Bauteil_6.BT_6_Y_Achse,Bauteil.Stempelanlage_BT.Bauteil_6.BT_6_Z_Achse
  Bus Selector13 : BusSelector  OutputSignals=Bauteil.Stempelanlage_BT.Bauteil_7.BT_7_X_Achse,Bauteil.Stempelanlage_BT.Bauteil_7.BT_7_Y_Achse,Bauteil.Stempelanlage_BT.Bauteil_7.BT_7_Z_Achse
  Bus Selector14 : BusSelector  OutputSignals=Bauteil.Stempelanlage_BT.Bauteil_8.BT_8_X_Achse,Bauteil.Stempelanlage_BT.Bauteil_8.BT_8_Y_Achse,Bauteil.Stempelanlage_BT.Bauteil_8.BT_8_Z_Achse
  Bus Selector15 : BusSelector  OutputSignals=Bauteil.Stempelanlage_BT.Bauteil_9.BT_9_X_Achse,Bauteil.Stempelanlage_BT.Bauteil_9.BT_9_Y_Achse,Bauteil.Stempelanlage_BT.Bauteil_9.BT_9_Z_Achse
  Bus Selector16 : BusSelector  OutputSignals=Eingaenge.Bauteile.BT_Sieben
  Bus Selector17 : BusSelector  OutputSignals=Eingaenge.Bauteile.BT_Acht
  Bus Selector18 : BusSelector  OutputSignals=Eingaenge.Bauteile.BT_Neun
  Bus Selector2 : BusSelector  OutputSignals=Eingaenge.Bauteile.BT_Eins
  Bus Selector3 : BusSelector  OutputSignals=Bauteil.Stempelanlage_BT.Bauteil_1.BT_1_X_Achse,Bauteil.Stempelanlage_BT.Bauteil_1.BT_1_Y_Achse,Bauteil.Stempelanlage_BT.Bauteil_1.BT_1_Z_Achse
  Bus Selector4 : BusSelector  OutputSignals=Eingaenge.Bauteile.BT_Zwei
  Bus Selector5 : BusSelector  OutputSignals=Eingaenge.Bauteile.BT_Drei
  Bus Selector6 : BusSelector  OutputSignals=Eingaenge.Bauteile.BT_Vier
  Bus Selector7 : BusSelector  OutputSignals=Eingaenge.Bauteile.BT_Fuenf
  Bus Selector8 : BusSelector  OutputSignals=Eingaenge.Bauteile.BT_Sechs
  Bus Selector9 : BusSelector  OutputSignals=Bauteil.Stempelanlage_BT.Bauteil_3.BT_3_X_Achse,Bauteil.Stempelanlage_BT.Bauteil_3.BT_3_Y_Achse,Bauteil.Stempelanlage_BT.Bauteil_3.BT_3_Z_Achse
  Compare To Constant{,13..17,60..62} (9 alike) : simulink/Logic and Bit Operations/Compare To Constant  relop===  const=1  OutDataTypeStr=boolean
  Compare To Constant{1,7,21,27,33,39,45,51,57} (9 alike) : simulink/Logic and Bit Operations/Compare To Constant  relop=<=  const=0.5  OutDataTypeStr=boolean
  Compare To Constant{4,10,18,24,30,36,42,48,54} (9 alike) : simulink/Logic and Bit Operations/Compare To Constant  relop=<=  const=-3.3  OutDataTypeStr=boolean
  Compare To Constant{5,11,19,25,31,37,43,49,55} (9 alike) : simulink/Logic and Bit Operations/Compare To Constant  relop=>=  const=-3.7  OutDataTypeStr=boolean
  Compare To Constant{6,12,20,26,32,38,44,50,56} (9 alike) : simulink/Logic and Bit Operations/Compare To Constant  relop=>=  const=-0.5  OutDataTypeStr=boolean
  Compare To Constant{2,8,22,28,34,40,46,52,58} (9 alike) : simulink/Logic and Bit Operations/Compare To Constant  relop=>=  const=0.5  OutDataTypeStr=boolean
  Compare To Constant{3,9,23,29,35,41,47,53,59} (9 alike) : simulink/Logic and Bit Operations/Compare To Constant  relop=<=  const=0.9  OutDataTypeStr=boolean
  Constant{,2,4,6,8,10,12,14,16} (9 alike) : Constant  Value=0
  Constant{1,3,5,7,9,11,13,15,17} (9 alike) : Constant
  Display{,1..4} (5 alike) : Display
  Logical Operator{,2..4,6..8,10..14,17..19,21..23,25..27,29..31,33..35,37..39,41..46} (36 alike) : Logic  AllPortsSameDT=off  OutDataTypeStr=boolean
  Logical Operator{1,5,16,20,24,28,32,36,40} (9 alike) : Logic  Inputs=3  AllPortsSameDT=off  OutDataTypeStr=boolean
  Logical Operator15 : Logic  Inputs=9  AllPortsSameDT=off  OutDataTypeStr=boolean
  Logical Operator9 : Logic  Operator=OR  Inputs=9  AllPortsSameDT=off  OutDataTypeStr=boolean
  Switch{1..9} (9 alike) : Switch  Threshold=1
  Sensor_Band_BT_Vorhanden : Outport
  Sensor_Band_Hell_1 : Outport  Port=2
  wires:
  Bus Selector3/2 -> Compare To Constant2/1, Compare To Constant3/1  "<BT_1_Y_Achse>"
  Compare To Constant2/1 -> Logical Operator3/1
  Compare To Constant3/1 -> Logical Operator3/2
  Logical Operator3/1 -> Logical Operator1/2
  Bus Selector3/3 -> Compare To Constant4/1, Compare To Constant5/1  "<BT_1_Z_Achse>"
  Compare To Constant4/1 -> Logical Operator2/1
  Compare To Constant5/1 -> Logical Operator2/2
  Logical Operator2/1 -> Logical Operator1/3
  Bus Selector3/1 -> Compare To Constant1/1, Compare To Constant6/1  "<BT_1_X_Achse>"
  Compare To Constant1/1 -> Logical Operator4/1
  Compare To Constant6/1 -> Logical Operator4/2
  Logical Operator4/1 -> Logical Operator1/1
  Bus Selector1/2 -> Compare To Constant8/1, Compare To Constant9/1  "<BT_2_Y_Achse>"
  Compare To Constant8/1 -> Logical Operator7/1
  Compare To Constant9/1 -> Logical Operator7/2
  Logical Operator7/1 -> Logical Operator5/2
  Logical Operator5/1 -> Logical Operator9/2, Display1/1, Logical Operator10/1
  Bus Selector1/3 -> Compare To Constant11/1, Compare To Constant10/1  "<BT_2_Z_Achse>"
  Compare To Constant10/1 -> Logical Operator6/1
  Compare To Constant11/1 -> Logical Operator6/2
  Logical Operator6/1 -> Logical Operator5/3
  Bus Selector1/1 -> Compare To Constant7/1, Compare To Constant12/1  "<BT_2_X_Achse>"
  Compare To Constant7/1 -> Logical Operator8/1
  Compare To Constant12/1 -> Logical Operator8/2
  Logical Operator8/1 -> Logical Operator5/1
  Logical Operator9/1 -> Sensor_Band_BT_Vorhanden/1
  Logical Operator1/1 -> Logical Operator9/1, Logical Operator/1
  Bus Selector2/1 -> Compare To Constant/1  "<BT_Eins>"
  Compare To Constant/1 -> Logical Operator/2
  Logical Operator/1 -> Switch6/2
  Constant/1 -> Switch6/1
  Constant1/1 -> Switch6/3
  Logical Operator10/1 -> Display3/1, Switch3/2
  Constant2/1 -> Switch3/1
  Constant3/1 -> Switch3/3
  Logical Operator11/1 -> Switch2/2
  Constant4/1 -> Switch2/1
  Constant5/1 -> Switch2/3
  Logical Operator12/1 -> Switch1/2
  Constant6/1 -> Switch1/1
  Constant7/1 -> Switch1/3
  Logical Operator13/1 -> Switch5/2
  Constant8/1 -> Switch5/1
  Constant9/1 -> Switch5/3
  Logical Operator14/1 -> Switch4/2
  Constant10/1 -> Switch4/1
  Constant11/1 -> Switch4/3
  Bus Selector4/1 -> Compare To Constant13/1  "<BT_Zwei>"
  Compare To Constant13/1 -> Display2/1, Logical Operator10/2
  Bus Selector5/1 -> Compare To Constant14/1  "<BT_Drei>"
  Compare To Constant14/1 -> Logical Operator11/2
  Bus Selector6/1 -> Compare To Constant15/1  "<BT_Vier>"
  Compare To Constant15/1 -> Logical Operator12/2
  Bus Selector7/1 -> Compare To Constant16/1  "<BT_Fuenf>"
  Compare To Constant16/1 -> Logical Operator13/2
  Bus Selector8/1 -> Compare To Constant17/1  "<BT_Sechs>"
  Compare To Constant17/1 -> Logical Operator14/2
  Switch6/1 -> Logical Operator15/1
  Switch3/1 -> Display/1, Logical Operator15/2
  Switch2/1 -> Logical Operator15/3
  Switch1/1 -> Logical Operator15/4
  Switch5/1 -> Logical Operator15/5
  Switch4/1 -> Logical Operator15/6
  Logical Operator15/1 -> Display4/1, Sensor_Band_Hell_1/1
  Bus Selector9/2 -> Compare To Constant22/1, Compare To Constant23/1  "<BT_3_Y_Achse>"
  Compare To Constant22/1 -> Logical Operator18/1
  Compare To Constant23/1 -> Logical Operator18/2
  Logical Operator18/1 -> Logical Operator16/2
  Bus Selector9/3 -> Compare To Constant19/1, Compare To Constant18/1  "<BT_3_Z_Achse>"
  Compare To Constant18/1 -> Logical Operator17/1
  Compare To Constant19/1 -> Logical Operator17/2
  Logical Operator17/1 -> Logical Operator16/3
  Bus Selector9/1 -> Compare To Constant21/1, Compare To Constant20/1  "<BT_3_X_Achse>"
  Compare To Constant21/1 -> Logical Operator19/1
  Compare To Constant20/1 -> Logical Operator19/2
  Logical Operator19/1 -> Logical Operator16/1
  Bus Selector10/2 -> Compare To Constant28/1, Compare To Constant29/1  "<BT_4_Y_Achse>"
  Compare To Constant28/1 -> Logical Operator22/1
  Compare To Constant29/1 -> Logical Operator22/2
  Logical Operator22/1 -> Logical Operator20/2
  Bus Selector10/3 -> Compare To Constant25/1, Compare To Constant24/1  "<BT_4_Z_Achse>"
  Compare To Constant24/1 -> Logical Operator21/1
  Compare To Constant25/1 -> Logical Operator21/2
  Logical Operator21/1 -> Logical Operator20/3
  Bus Selector10/1 -> Compare To Constant27/1, Compare To Constant26/1  "<BT_4_X_Achse>"
  Compare To Constant27/1 -> Logical Operator23/1
  Compare To Constant26/1 -> Logical Operator23/2
  Logical Operator23/1 -> Logical Operator20/1
  Bus Selector11/2 -> Compare To Constant34/1, Compare To Constant35/1  "<BT_5_Y_Achse>"
  Compare To Constant34/1 -> Logical Operator26/1
  Compare To Constant35/1 -> Logical Operator26/2
  Logical Operator26/1 -> Logical Operator24/2
  Bus Selector11/3 -> Compare To Constant31/1, Compare To Constant30/1  "<BT_5_Z_Achse>"
  Compare To Constant30/1 -> Logical Operator25/1
  Compare To Constant31/1 -> Logical Operator25/2
  Logical Operator25/1 -> Logical Operator24/3
  Bus Selector11/1 -> Compare To Constant33/1, Compare To Constant32/1  "<BT_5_X_Achse>"
  Compare To Constant33/1 -> Logical Operator27/1
  Compare To Constant32/1 -> Logical Operator27/2
  Logical Operator27/1 -> Logical Operator24/1
  Bus Selector12/2 -> Compare To Constant40/1, Compare To Constant41/1  "<BT_6_Y_Achse>"
  Compare To Constant40/1 -> Logical Operator30/1
  Compare To Constant41/1 -> Logical Operator30/2
  Logical Operator30/1 -> Logical Operator28/2
  Bus Selector12/3 -> Compare To Constant37/1, Compare To Constant36/1  "<BT_6_Z_Achse>"
  Compare To Constant36/1 -> Logical Operator29/1
  Compare To Constant37/1 -> Logical Operator29/2
  Logical Operator29/1 -> Logical Operator28/3
  Bus Selector12/1 -> Compare To Constant39/1, Compare To Constant38/1  "<BT_6_X_Achse>"
  Compare To Constant39/1 -> Logical Operator31/1
  Compare To Constant38/1 -> Logical Operator31/2
  Logical Operator31/1 -> Logical Operator28/1
  Logical Operator16/1 -> Logical Operator9/3, Logical Operator11/1
  Logical Operator24/1 -> Logical Operator9/5, Logical Operator13/1
  Logical Operator28/1 -> Logical Operator9/6, Logical Operator14/1
  Logical Operator20/1 -> Logical Operator9/4, Logical Operator12/1
  Bus Selector13/2 -> Compare To Constant46/1, Compare To Constant47/1  "<BT_7_Y_Achse>"
  Compare To Constant46/1 -> Logical Operator34/1
  Compare To Constant47/1 -> Logical Operator34/2
  Logical Operator34/1 -> Logical Operator32/2
  Bus Selector13/3 -> Compare To Constant43/1, Compare To Constant42/1  "<BT_7_Z_Achse>"
  Compare To Constant42/1 -> Logical Operator33/1
  Compare To Constant43/1 -> Logical Operator33/2
  Logical Operator33/1 -> Logical Operator32/3
  Bus Selector13/1 -> Compare To Constant45/1, Compare To Constant44/1  "<BT_7_X_Achse>"
  Compare To Constant45/1 -> Logical Operator35/1
  Compare To Constant44/1 -> Logical Operator35/2
  Logical Operator35/1 -> Logical Operator32/1
  Bus Selector14/2 -> Compare To Constant52/1, Compare To Constant53/1  "<BT_8_Y_Achse>"
  Compare To Constant52/1 -> Logical Operator38/1
  Compare To Constant53/1 -> Logical Operator38/2
  Logical Operator38/1 -> Logical Operator36/2
  Bus Selector14/3 -> Compare To Constant49/1, Compare To Constant48/1  "<BT_8_Z_Achse>"
  Compare To Constant48/1 -> Logical Operator37/1
  Compare To Constant49/1 -> Logical Operator37/2
  Logical Operator37/1 -> Logical Operator36/3
  Bus Selector14/1 -> Compare To Constant51/1, Compare To Constant50/1  "<BT_8_X_Achse>"
  Compare To Constant51/1 -> Logical Operator39/1
  Compare To Constant50/1 -> Logical Operator39/2
  Logical Operator39/1 -> Logical Operator36/1
  Bus Selector15/2 -> Compare To Constant58/1, Compare To Constant59/1  "<BT_9_Y_Achse>"
  Compare To Constant58/1 -> Logical Operator42/1
  Compare To Constant59/1 -> Logical Operator42/2
  Logical Operator42/1 -> Logical Operator40/2
  Bus Selector15/3 -> Compare To Constant55/1, Compare To Constant54/1  "<BT_9_Z_Achse>"
  Compare To Constant54/1 -> Logical Operator41/1
  Compare To Constant55/1 -> Logical Operator41/2
  Logical Operator41/1 -> Logical Operator40/3
  Bus Selector15/1 -> Compare To Constant57/1, Compare To Constant56/1  "<BT_9_X_Achse>"
  Compare To Constant57/1 -> Logical Operator43/1
  Compare To Constant56/1 -> Logical Operator43/2
  Logical Operator43/1 -> Logical Operator40/1
  Logical Operator44/1 -> Switch7/2
  Constant12/1 -> Switch7/1
  Constant13/1 -> Switch7/3
  Bus Selector16/1 -> Compare To Constant60/1  "<BT_Sieben>"
  Compare To Constant60/1 -> Logical Operator44/2
  Switch7/1 -> Logical Operator15/7
  Inputs/1 -> Bus Selector9/1, Bus Selector10/1, Bus Selector11/1, Bus Selector12/1, Bus Selector13/1, Bus Selector14/1, Bus Selector15/1, Bus Selector18/1, Bus Selector17/1, Bus Selector16/1, Bus Selector8/1, Bus Selector7/1, Bus Selector6/1, Bus Selector5/1, Bus Selector4/1, Bus Selector2/1, Bus Selector1/1, Bus Selector3/1
  Logical Operator45/1 -> Switch8/2
  Constant14/1 -> Switch8/1
  Constant15/1 -> Switch8/3
  Bus Selector17/1 -> Compare To Constant61/1  "<BT_Acht>"
  Compare To Constant61/1 -> Logical Operator45/2
  Switch8/1 -> Logical Operator15/8
  Logical Operator46/1 -> Switch9/2
  Constant16/1 -> Switch9/1
  Constant17/1 -> Switch9/3
  Bus Selector18/1 -> Compare To Constant62/1  "<BT_Neun>"
  Compare To Constant62/1 -> Logical Operator46/2
  Switch9/1 -> Logical Operator15/9
  Logical Operator32/1 -> Logical Operator44/1, Logical Operator9/7
  Logical Operator36/1 -> Logical Operator45/1, Logical Operator9/8
  Logical Operator40/1 -> Logical Operator46/1, Logical Operator9/9
